simulink model "modeloLQR"  (R2018b)
settings: Solver=VariableStepAuto  StartTime=0.0  StopTime=30  RelTol=1e-3
values from neighbouring files (symbols this model uses):
  A = [0      1              0           0 ... (first row only)    [intento.m]    (also in prueba.m; task.m = [0,                     0,          0,                      ; task_LQR.m = [             0, 1, 0,                   0; task_PID.m = [             0, 1, 0,                   0)
  B = [     0 ... (first row only)    [intento.m]    (also in prueba.m; task.m = [0; 1/(L*mc); 0; 1/mc]; task_LQR.m = [0; -M*L/p; 0; (I+M*L^2)/p]; task_PID.m = [0; (-L*m*p1)/(M+m); 0; p2])
  K = lqr(A,B,Q,R)    [intento.m]    (also in prueba.m = K*C; task.m = [K1; K2; K3; K4]; task_LQR.m = [K_angulo; K_rate; K_pos; K_vel]; task_PID.m = [K_angulo; K_rate; K_pos; K_vel])
  T1 = diag([deg2rad; deg2rad; rad2m; rad2m])    [intento.m]    (also in task_PID.m = diag([deg2rad; deg2rad; 1; 1]))
  T2 = diag([rad2deg; rad2deg; 1; 1])    [task_PID.m]
  x0 = [0.2; 0; 0; 0]    [intento.m]    (also in prueba.m = [0; 0; 0.2; 0]; task.m = [5*pi/180; 0; 0; 0]; task_LQR.m; task_PID.m = [5*deg2rad; 0; 0; 0])
settings Model: Creator=vuvux  LastModifiedBy=vuvux

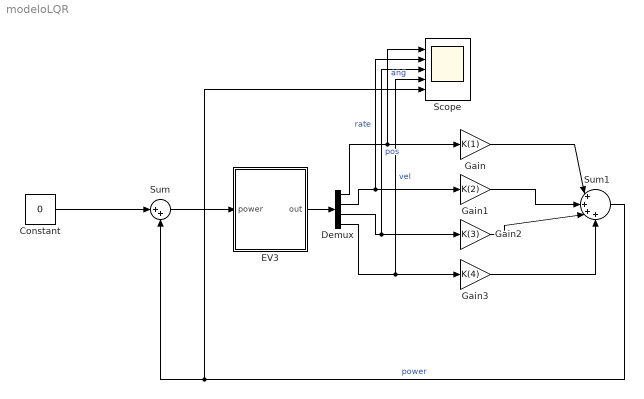
== system modeloLQR ==
  Constant : Constant  Value=0
  Demux : Demux
  "EV3 " : Subsystem
  Gain : Gain  Gain=K(1)
  Gain1 : Gain  Gain=K(2)
  Gain2 : Gain  Gain=K(3)
  Gain3 : Gain  Gain=K(4)
  Scope : Scope  NumInputPorts=5
  Sum : Sum  Inputs=|++
  Sum1 : Sum  Inputs=|++++
  wires:
  Constant/1 -> Sum/1
  Sum1/1 -> Scope/5, Sum/2  "power"
  Sum/1 -> "EV3 "/1(power)
  Gain/1 -> Sum1/1
  Gain1/1 -> Sum1/2
  Gain2/1 -> Sum1/3
  Gain3/1 -> Sum1/4
  Demux/2 -> Scope/2, Gain1/1  "rate"
  "EV3 "/1(out) -> Demux/1
  Demux/1 -> Scope/1, Gain/1  "ang"
  Demux/3 -> Scope/3, Gain2/1  "pos"
  Demux/4 -> Scope/4, Gain3/1  "vel"

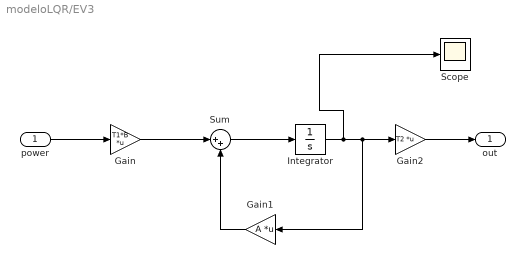
== system modeloLQR/EV3  ==
  power : Inport
  Gain : Gain  Gain=T1*B  Multiplication=Matrix(K*u)
  Gain1 : Gain  Gain=A  Multiplication=Matrix(K*u)
  Gain2 : Gain  Gain=T2  Multiplication=Matrix(K*u) (u vector)
  Integrator : Integrator  InitialCondition=x0
  Scope : Scope
  Sum : Sum  Inputs=|++
  out : Outport
  wires:
  Gain1/1 -> Sum/2
  Gain/1 -> Sum/1
  Sum/1 -> Integrator/1
  power/1 -> Gain/1
  Integrator/1 -> Scope/1, Gain2/1, Gain1/1
  Gain2/1 -> out/1
